simulink model "task1b_1"  (R2019a)
settings: Solver=VariableStepAuto  StartTime=0.0  StopTime=10.0  RelTol=1e-3
settings Model: Creator=Artem  LastModifiedBy=Artem

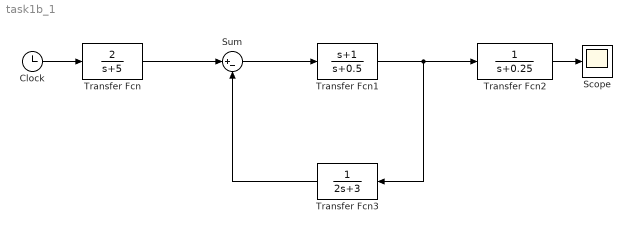
== system task1b_1 ==
  Clock : Clock
  Scope : Scope
  Sum : Sum  Inputs=|+-
  Transfer Fcn : TransferFcn  Numerator=[2]  Denominator=[1 5]
  Transfer Fcn1 : TransferFcn  Numerator=[1 1]  Denominator=[1 0.5]
  Transfer Fcn2 : TransferFcn  Denominator=[1 0.25]
  Transfer Fcn3 : TransferFcn  Denominator=[2 3]
  wires:
  Transfer Fcn/1 -> Sum/1
  Sum/1 -> Transfer Fcn1/1
  Transfer Fcn1/1 -> Transfer Fcn3/1, Transfer Fcn2/1
  Transfer Fcn3/1 -> Sum/2
  Transfer Fcn2/1 -> Scope/1
  Clock/1 -> Transfer Fcn/1
